simulink model "bb_linear_model"  (R2020a)
settings: Solver=VariableStepAuto  StartTime=0.0  StopTime=300  RelTol=1e-3
values from neighbouring files (symbols this model uses):
  A = double(subs(A_hat, [m R g Jb], [.5 .015 9.8 9.99e-3]))    [beam_and_ball_linear.m]
  B = double(B_hat)    [beam_and_ball_linear.m]
  C = [1 0 0 0]    [beam_and_ball_linear.m]
  l_lqr_d = dlqr(Ad', Cd', Q*1.2, R)    [beam_and_ball_linear.m]
  Ts = .1    (= 0.1)    [beam_and_ball_linear.m]
  x0 = [0 0 0 0]    [beam_and_ball_linear.m]
undefined symbols (not defined in the file or in its folder): Ad, Bd, Cd, k_lqr_d
settings Model: Creator=mehdikoochak  LastModifiedBy=mehdikoochak

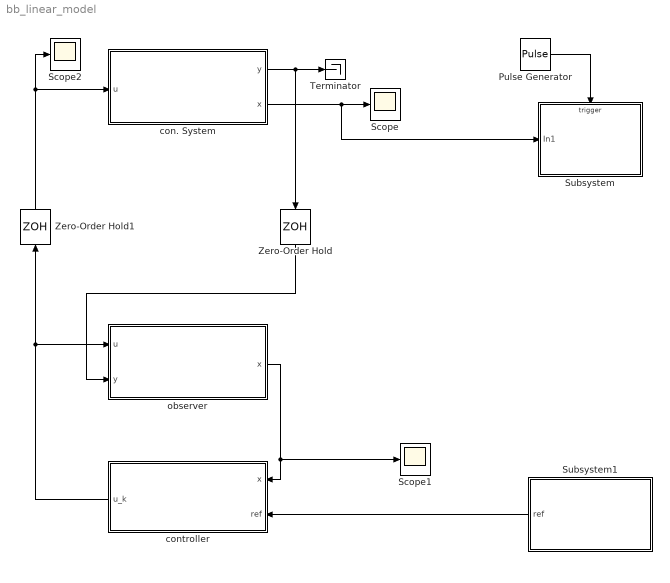
== system bb_linear_model ==
  Pulse Generator : DiscretePulseGenerator  PulseType=Time based  Period=Ts  PulseWidth=50
  Scope : Scope
  Scope1 : Scope
  Scope2 : Scope
  Subsystem : Subsystem
  Subsystem1 : Subsystem
  Terminator : Terminator
  Zero-Order Hold : ZeroOrderHold  SampleTime=Ts
  Zero-Order Hold1 : ZeroOrderHold  SampleTime=Ts
  con. System : Subsystem
  controller : Subsystem
  observer : Subsystem
  wires:
  con. System/2(x) -> Subsystem/1(In1), Scope/1
  con. System/1(y) -> Terminator/1, Zero-Order Hold/1
  controller/1(u_k) -> observer/1(u), Zero-Order Hold1/1
  Subsystem1/1(ref) -> controller/2(ref)
  Zero-Order Hold1/1 -> Scope2/1, con. System/1(u)
  Zero-Order Hold/1 -> observer/2(y)
  observer/1(x) -> controller/1(x), Scope1/1
  Pulse Generator/1 -> Subsystem/Trigger

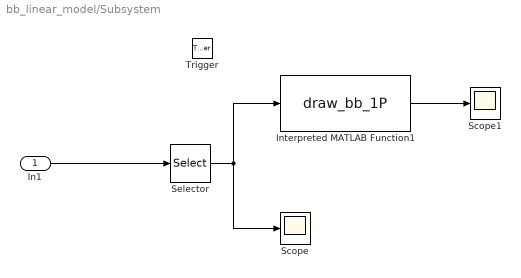
== system bb_linear_model/Subsystem ==
  In1 : Inport
  Trigger : TriggerPort  VariantControl=Variant  PortDimensions=1
  Interpreted MATLAB Function1 : MATLABFcn  MATLABFcn=draw_bb_1P  OutputDimensions=1
  Scope : Scope
  Scope1 : Scope
  Selector : Selector  InputPortWidth=4  IndexOptions=Index vector (dialog)  Indices=[1 3]  OutputSizes=1
  wires:
  In1/1 -> Selector/1
  Selector/1 -> Interpreted MATLAB Function1/1, Scope/1
  Interpreted MATLAB Function1/1 -> Scope1/1

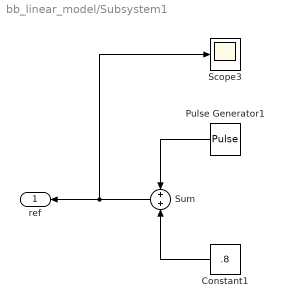
== system bb_linear_model/Subsystem1 ==
  Constant1 : Constant  Value=.8
  Pulse Generator1 : DiscretePulseGenerator  PulseType=Time based  Amplitude=-.8  Period=20  PulseWidth=50
  Scope3 : Scope
  Sum : Sum
  ref : Outport
  wires:
  Pulse Generator1/1 -> Sum/1
  Constant1/1 -> Sum/2
  Sum/1 -> ref/1, Scope3/1

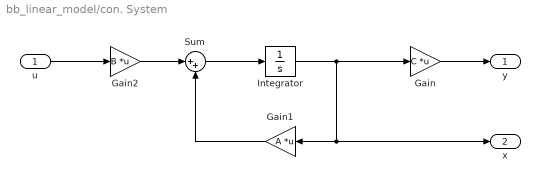
== system bb_linear_model/con. System ==
  u : Inport
  Gain : Gain  Gain=C  Multiplication=Matrix(K*u)
  Gain1 : Gain  Gain=A  Multiplication=Matrix(K*u)
  Gain2 : Gain  Gain=B  Multiplication=Matrix(K*u)
  Integrator : Integrator  InitialCondition=x0
  Sum : Sum  Inputs=|++
  y : Outport
  x : Outport  Port=2
  wires:
  Gain1/1 -> Sum/2
  u/1 -> Gain2/1
  Gain/1 -> y/1
  Gain2/1 -> Sum/1
  Sum/1 -> Integrator/1
  Integrator/1 -> Gain/1, Gain1/1, x/1

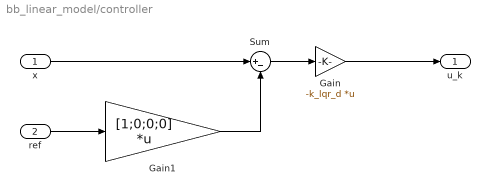
== system bb_linear_model/controller ==
  x : Inport
  ref : Inport  Port=2
  Gain : Gain  Gain=-k_lqr_d  Multiplication=Matrix(K*u)
  Gain1 : Gain  Gain=[1;0;0;0]  Multiplication=Matrix(K*u)
  Sum : Sum  Inputs=|+-
  u_k : Outport
  wires:
  Gain/1 -> u_k/1
  Gain1/1 -> Sum/2
  ref/1 -> Gain1/1
  x/1 -> Sum/1
  Sum/1 -> Gain/1

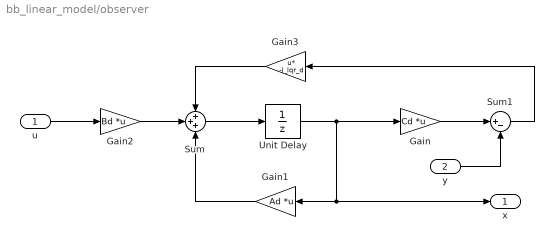
== system bb_linear_model/observer ==
  u : Inport
  y : Inport  Port=2
  Gain : Gain  Gain=Cd  Multiplication=Matrix(K*u)
  Gain1 : Gain  Gain=Ad  Multiplication=Matrix(K*u)
  Gain2 : Gain  Gain=Bd  Multiplication=Matrix(K*u)
  Gain3 : Gain  Gain=-l_lqr_d  Multiplication=Matrix(u*K)
  Sum : Sum  Inputs=+++
  Sum1 : Sum  Inputs=|+-
  Unit Delay : UnitDelay  SampleTime=Ts  HasFrameUpgradeWarning=on
  x : Outport
  wires:
  u/1 -> Gain2/1
  Gain/1 -> Sum1/1
  Sum/1 -> Unit Delay/1
  Unit Delay/1 -> Gain/1, Gain1/1, x/1
  Gain1/1 -> Sum/3
  Gain2/1 -> Sum/2
  Gain3/1 -> Sum/1
  y/1 -> Sum1/2
  Sum1/1 -> Gain3/1
